simulink model "voltage_sensors_calibration"  (R2022b)
settings: Solver=VariableStepAuto  StartTime=0.0  StopTime=10.0  RelTol=1e-3  EnableMultiTasking=on
libraries: c2802xlib x3, spsFirstOrderFilterLib x3
settings Model: Creator=menna  LastModifiedBy=menna
settings SolverCC: PositivePriorityOrder=on
settings OptimizationCC: EnhancedBackFolding=on  PassReuseOutputArgsAs=Individual arguments  ZeroExternalMemoryAtStartup=off  ZeroInternalMemoryAtStartup=off  MaxStackSize=64  OptimizeBlockOrder=speed  DifferentSizesBufferReuse=on  OptimizationCustomize=off  EfficientTunableParamExpr=on
settings DebuggingCC: ParameterTunabilityLossMsg=error
settings HardwareCC: ProdBitPerChar=16  ProdBitPerInt=16  ProdBitPerPointer=32  ProdBitPerSizeT=32  ProdBitPerPtrDiffT=32  ProdLargestAtomicInteger=Integer  ProdLargestAtomicFloat=None  ProdWordSize=16  ProdHWDeviceType=Texas Instruments->C2000  HardwareBoardFeatureSet=SoCBlockset
settings ModelReferenceCC: ModelReferenceNumInstancesAllowed=Single
settings SFSimCC: MATLABDynamicMemAlloc=off
settings RTWCC: Description=Embedded Coder  SystemTargetFile=ert.tlc  HardwareBoard=TI Delfino F28379D LaunchPad  TLCOptions=-aInlineSetEventsForThisBaseRateFcn=TLC_FALSE -aSuppressMultiTaskScheduler=TLC_FALSE -aRateBasedStepFcn=1  TemplateMakefile=ert_default_tmf
settings CodeAppCC: ForceParamTrailComments=on  IgnoreCustomStorageClasses=off  OperatorAnnotations=on  SimulinkDataObjDesc=on  SFDataObjDesc=on  InsertBlockDesc=on
settings ERTTargetCC: ExtModeMexFile=TIC2000ExternalModeOpen  ExtModeIntrfLevel=Level2 - Open

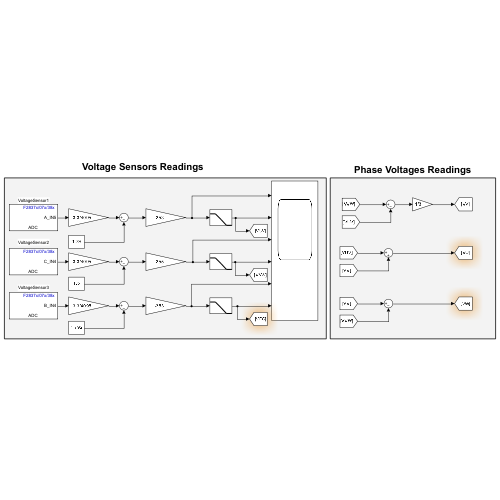
[thumbnail: Simulink's stored preview of the top-level diagram]
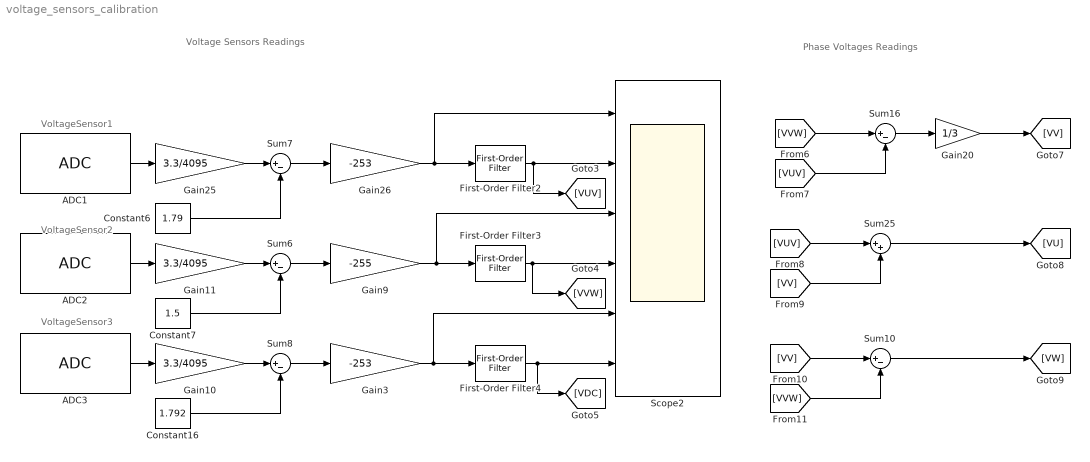
== system voltage_sensors_calibration ==
  note: Phase Voltages Readings
  note: VoltageSensor2
  note: VoltageSensor3
  note: Voltage Sensors Readings
  note: VoltageSensor1
  ADC1 : c2802xlib/ADC  blkParamProc=C2000_Type4  ADCModule=A  samplingMode=Single sample mode  ADCResolution=12-bit (Single-ended input)  useSOC1=SOC0  useSOC2=SOC0_SOC1  SOCAcquisitionWindow=15  SOCTriggerSource=Software  SOCInterruptTrigger=No ADCINT  Ts=1e-4  dType=uint16  postInterrupt=off  interruptSel=ADCINT1  ADCINTContinuous=on  endma=off  chdma=1  conv1=ADCINA0  conv2=ADCINA0 and ADCINB0  conv1_Type4=ADCIN5  conv2_Type4=ADCIN0 and ADCIN1
      settings: LibrarySourceBlock=c2837xDlib/ADC
  ADC2 : c2802xlib/ADC  blkParamProc=C2000_Type4  ADCModule=C  samplingMode=Single sample mode  ADCResolution=12-bit (Single-ended input)  useSOC1=SOC2  useSOC2=SOC0_SOC1  SOCAcquisitionWindow=15  SOCTriggerSource=Software  SOCInterruptTrigger=No ADCINT  Ts=1e-4  dType=uint16  postInterrupt=off  interruptSel=ADCINT1  ADCINTContinuous=on  endma=off  chdma=1  conv1=ADCINA0  conv2=ADCINA0 and ADCINB0  conv1_Type4=ADCIN4  conv2_Type4=ADCIN0 and ADCIN1
      settings: LibrarySourceBlock=c2837xDlib/ADC
  ADC3 : c2802xlib/ADC  blkParamProc=C2000_Type4  ADCModule=B  samplingMode=Single sample mode  ADCResolution=12-bit (Single-ended input)  useSOC1=SOC1  useSOC2=SOC0_SOC1  SOCAcquisitionWindow=15  SOCTriggerSource=Software  SOCInterruptTrigger=No ADCINT  Ts=0.001  dType=uint16  postInterrupt=off  interruptSel=ADCINT1  ADCINTContinuous=on  endma=off  chdma=1  conv1=ADCINA0  conv2=ADCINA0 and ADCINB0  conv1_Type4=ADCIN4  conv2_Type4=ADCIN0 and ADCIN1
      settings: LibrarySourceBlock=c2837xDlib/ADC
  Constant16 : Constant  Value=1.792  SampleTime=-1
  Constant6 : Constant  Value=1.79  SampleTime=-1
  Constant7 : Constant  Value=1.5  SampleTime=-1
  First-Order Filter2 : spsFirstOrderFilterLib/First-Order Filter  FilterType=Lowpass  Tc=1/250  Ts=1/5000  Initialize=off  Vac_Init=[0, 0, 60]  Vdc_Init=0  PlotResponse=off  FreqRange="[0,  200,  1]"
  First-Order Filter3 : spsFirstOrderFilterLib/First-Order Filter  FilterType=Lowpass  Tc=1/250  Ts=1/5000  Initialize=off  Vac_Init=[0, 0, 60]  Vdc_Init=0  PlotResponse=off  FreqRange="[0,  200,  1]"
  First-Order Filter4 : spsFirstOrderFilterLib/First-Order Filter  FilterType=Lowpass  Tc=1/250  Ts=1/5000  Initialize=off  Vac_Init=[0, 0, 60]  Vdc_Init=0  PlotResponse=off  FreqRange="[0,  200,  1]"
  Gain10 : Gain  Gain=3.3/4095
  Gain11 : Gain  Gain=3.3/4095
  Gain20 : Gain  Gain=1/3
  Gain25 : Gain  Gain=3.3/4095
  Gain26 : Gain  Gain=-253
  Gain3 : Gain  Gain=-253
  Gain9 : Gain  Gain=-255
  Scope2 : Scope  NumInputPorts=6
  Sum{6..8,10,16} (5 alike) : Sum  Inputs=|+-
  Sum25 : Sum  Inputs=|++
  wires:
  Sum16/1 -> Gain20/1
  ADC1/1 -> Gain25/1
  [VV] -> Sum10/1
  [VVW] -> Sum10/2
  Constant6/1 -> Sum7/2
  Gain11/1 -> Sum6/1
  [VVW] -> Sum16/1
  First-Order Filter2/1 -> Scope2/2, [VUV]
  Gain9/1 -> Scope2/3, First-Order Filter3/1
  Sum8/1 -> Gain3/1
  Gain25/1 -> Sum7/1
  Gain3/1 -> First-Order Filter4/1, Scope2/5
  Constant7/1 -> Sum6/2
  Sum6/1 -> Gain9/1
  Sum25/1 -> [VU]
  ADC2/1 -> Gain11/1
  Gain26/1 -> Scope2/1, First-Order Filter2/1
  Gain20/1 -> [VV]
  First-Order Filter3/1 -> Scope2/4, [VVW]
  Constant16/1 -> Sum8/2
  Gain10/1 -> Sum8/1
  [VUV] -> Sum25/1
  Sum10/1 -> [VW]
  [VUV] -> Sum16/2
  [VV] -> Sum25/2
  First-Order Filter4/1 -> [VDC], Scope2/6
  ADC3/1 -> Gain10/1
  Sum7/1 -> Gain26/1
